simulink model "ssc_dcmtr_sl"  (R2022b)
settings: Solver=VariableStepAuto  StartTime=0.0  StopTime=10.0  RelTol=1e-3
model workspace (MAT data in the model file):
  J = 0.0946866703633
  K = 0.477771340295
  L = 0.000316454712175
  R = 4.99938152603
  Tbrk = 0.001
  Tcolumb = 0.001
  Ts = 0.01
  Tvis = 0.001
  b = 0.921434142151
libraries: fl_lib x6, nesl_utility x3, ee_lib x1
settings Model: Creator=smuckati  LastModifiedBy=smuckati
settings DebuggingCC: ParameterPrecisionLossMsg=none  UnconnectedInputMsg=warning  UnconnectedOutputMsg=warning  UnconnectedLineMsg=warning
settings ModelReferenceCC: EnableRefExpFcnMdlSchedulingChecks=on
settings RTWCC: DLArmComputeVersion=19.05

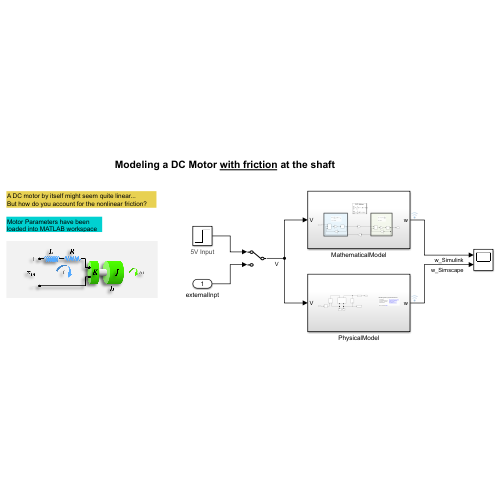
[thumbnail: Simulink's stored preview of the top-level diagram]
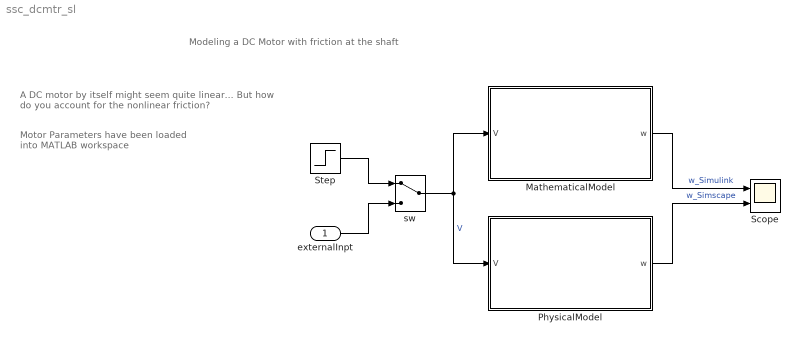
== system ssc_dcmtr_sl ==
  note: A DC motor by itself might seem quite linear...
      | But how do you account for the nonlinear friction?
  note: Modeling a DC Motor with friction at the shaft
  note: Motor Parameters have been loaded into MATLAB workspace
  externalInpt : Inport
  MathematicalModel : Subsystem
  PhysicalModel : Subsystem
  Scope : Scope  NumInputPorts=2
  Step : Step  Time=2  After=5  SampleTime=0
      settings: AttributesFormatString=5V Input
  sw : ManualSwitch
  wires:
  PhysicalModel/1(w) -> Scope/2  "w_Simscape"
  MathematicalModel/1(w) -> Scope/1  "w_Simulink"
  sw/1 -> PhysicalModel/1(V), MathematicalModel/1(V)  "V"
  externalInpt/1 -> sw/2
  Step/1 -> sw/1

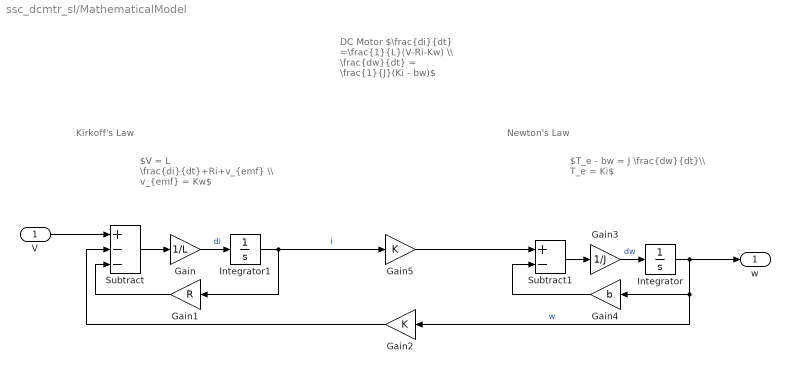
== system ssc_dcmtr_sl/MathematicalModel ==
  note: Newton's Law
  note: $T_e - bw = J \frac{dw}{dt}\\ T_e = Ki$
  note: Kirkoff's Law
  note: $V = L \frac{di}{dt}+Ri+v_{emf} \\ v_{emf} = Kw$
  note: DC Motor
      | $\frac{di}{dt} =\frac{1}{L}(V-Ri-Kw) \\ \frac{dw}{dt} = \frac{1}{J}(Ki - bw)$
  V : Inport
  Gain : Gain  Gain=1/L
  Gain1 : Gain  Gain=R
  Gain2 : Gain  Gain=K
  Gain3 : Gain  Gain=1/J
  Gain4 : Gain  Gain=b
  Gain5 : Gain  Gain=K
  Integrator : Integrator
  Integrator1 : Integrator
  Subtract : Sum  Inputs=+--
  Subtract1 : Sum  Inputs=+-
  w : Outport  VectorParamsAs1DForOutWhenUnconnected=off
  wires:
  Gain1/1 -> Subtract/3
  Integrator1/1 -> Gain5/1, Gain1/1  "i"
  Integrator/1 -> w/1, Gain2/1, Gain4/1  "w"
  Gain2/1 -> Subtract/2
  Subtract1/1 -> Gain3/1
  Gain3/1 -> Integrator/1  "dw"
  Gain4/1 -> Subtract1/2
  Gain5/1 -> Subtract1/1
  Subtract/1 -> Gain/1
  Gain/1 -> Integrator1/1  "di"
  V/1 -> Subtract/1

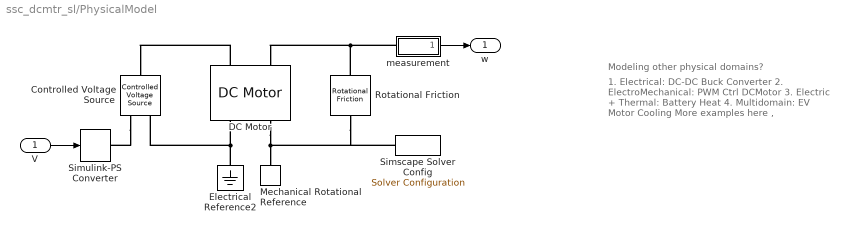
== system ssc_dcmtr_sl/PhysicalModel ==
  note: 1. Electrical: DC-DC Buck Converter
      | 2. ElectroMechanical: PWM Ctrl DCMotor
      | 3. Electric + Thermal: Battery Heat
      | 4. Multidomain: EV Motor Cooling
      |
      | More examples here ,
  note: Modeling other physical domains?
  V : Inport
  Controlled Voltage Source : fl_lib/Electrical/Electrical Sources/Controlled Voltage Source
  DC Motor : ee_lib/Electromechanical/Brushed Motors/DC Motor  field_option=ee.enum.field_option.pm  Rf=100 Ohm  Lf=1 H  Laf=0.15 H  If0=0 A  parameterization=ee.enum.dcparam_option.circuit_param  Ra=R Ohm  La=L H  emf_or_torque=ee.enum.emf_or_torque.ki  Kv=K V/(rad/s)  Ki=K N*m/A  T_stall=57/16 in*lbf  w_max=62.5 rpm  w_rated=1.5e+04 rpm  P_rated=0.08 W  V_rated=5 V  lam_param=ee.enum.lam_param.damping  i_noload=0 A  V_i_noload=1.5 V  J=J kg*m^2  lam=b N*m/(rad/s)  speed0=0 rpm  enable_fault_armature=simscape.enum.onoff.off  rev_faulted=1 / 3  G_faulted_armature=1e-5 S  fault_trigger_armature=ee.enum.faults.faultTrigger.temporal  t_fault_armature=1 s  max_permissible_current_armature=inf A  t_fail_on_current_armature=1 s  enable_fault_field=simscape.enum.onoff.off  G_faulted_field=1e-5 S  fault_trigger_field=ee.enum.faults.faultTrigger.temporal  t_fault_field=1 s  max_permissible_current_field=inf A  t_fail_on_current_field=1 s  fault_action=simscape.enum.assert.action.none  alpha=3.93e-3 1/K  Tmeas=25 degC  thermal_mass=100 J/K  initial_temperature=25 degC
  Electrical Reference2 : fl_lib/Electrical/Electrical Elements/Electrical Reference
  Mechanical Rotational Reference : fl_lib/Mechanical/Rotational Elements/Mechanical Rotational Reference
  Rotational Friction : fl_lib/Mechanical/Rotational Elements/Rotational Friction  brkwy_trq=Tbrk N*m  brkwy_vel=0.001 rad/s  Col_trq=Tcolumb N*m  visc_coef=Tvis N*m/(rad/s)  w_specify=off  w_priority=None  w=0 rad/s  w_nominal_specify=off  w_nominal_unit=rad/s  w_nominal_value=1  t_specify=off  t_priority=None  t=0 N*m  t_nominal_specify=off  t_nominal_unit=N*m  t_nominal_value=1
  Simscape Solver Config : nesl_utility/Solver Configuration  PhysicalDomain=network_engine_domain  SubClassName=solver  LeftPortType=input  RightPortType=generic  Tones=[]  Harmonics=[]  SimulateNoise=off  Profile=off  UseLocalSampling=off  EnableSwitchedLinearOptims=on  FrequencyDomain=off  UseCCode=off  RelTol=0.001  AbsTol=1e-06  MinStep=1e-09  ToWorkspace=off  RevertToSquareIcSolve=off  NumHomotopyIterations=100  PhasorMode=off  PhasorModeNumHarmonics=1  ConsistencySolver=NEWTON_XTOL_AFTER_FTOL  IndexReductionMethod=DerivativeReplacement  DoDC=off  ResidualTolerance=1e-9  ConsistencyTolSource=GLOBAL  ConsistencyAbsTol=0.001  ConsistencyRelTol=0.001  ConsistencyTolFactor=0.001  UseLocalSolver=off  LocalSolverChoice=NE_BACKWARD_EULER_ADVANCER  ResolveIndetEquations=on  FunctionEvalNumThread=1  LocalSolverSampleTime=0.00125  DoFixedCost=off  MaxNonlinIter=3  MaxModeIter=2  ComputeImpulses=off  ImpulseIterations=2  LinearAlgebra=Sparse  LinearAlgebraNumThread=0  EquationFormulation=NE_TIME_EF  DelaysMemoryBudget=1024  AutomaticFiltering=on  FilteringTimeConstant=0.001  PartitionStorageMethod=AS_NEEDED  PartitionMemoryBudget=1024  PartitionMethod=FAST
  Simulink-PS Converter : nesl_utility/Simulink-PS Converter  PhysicalDomain=network_engine_domain  SubClassName=ps_input  LeftPortType=input  RightPortType=output  PseudoPeriodic=off  Frequencies=[]  NoiseDistribution=none  NoiseParameters=[]  Unit=1  AffineConversion=off  FilteringAndDerivatives=zero  SimscapeFilterOrder=1  InputFilterTimeConstant=.001  UdotUserProvided=0
  measurement : Subsystem
      settings: PortSchema="{\"entries\":[{\"content\":{\"sides\":[{\"content\":{\"connectorIds\":[]},\"type\":\"ConnectorPlacement.EquallySpacedRectSide\",\"uuid\":\"abba8c98-b5a4-4c4c-8426-d04bb5bd8376\"},{\"content\":{\"connectorIds\":[],\"side\":\"RIGHT\"},\"type\":\"ConnectorPlacement.EquallySpacedRectSide\",\"uuid\":\"4c88a845-695e-489f-8958-399be31258ba\"},{\"content\":{\"connectorIds\":[\"LConn1\"],\"side\":\"TOP\"},\"type\":\"ConnectorPlacement.EquallySpacedRectSide\",\"uuid\":\"679bc764-0dc4-40d2-b029-a4ea74e3efc8\"},{\"content\":{\"connectorIds\":[\"Out1\"],\"side\":\"BOTTOM\"},\"type\":\"ConnectorPlacement.EquallySpacedRectSide\",\"uuid\":\"9fb1c662-f4af-4578-8c70-f395a6f7f535\"}]},\"type\":\"ConnectorPlacement.EquallySpacedConnector\",\"uuid\":\"424eb965-f1ce-46f3-b179-04fc10bc201b\"}],\"packageUris\":[\"http://schema.mathworks.com/mf0/Connector/R2020b\"],\"version\":\"1.0\"}"
      mask Display: disp('Sensor')
  w : Outport  VectorParamsAs1DForOutWhenUnconnected=off
  wires:
  V/1 -> Simulink-PS Converter/1
  measurement/1(ang_vel) -> w/1
  connections:
  Electrical Reference2/LConn1 -- Controlled Voltage Source/RConn2 -- DC Motor/RConn1
  Controlled Voltage Source/RConn1 -- Simulink-PS Converter/RConn1
  DC Motor/RConn2 -- Rotational Friction/RConn1 -- Simscape Solver Config/RConn1 -- Mechanical Rotational Reference/LConn1
  measurement/LConn1 -- Rotational Friction/LConn1 -- DC Motor/LConn2
  DC Motor/LConn1 -- Controlled Voltage Source/LConn1

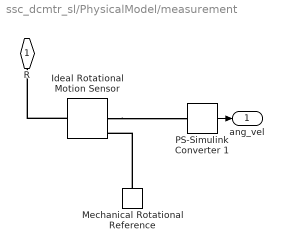
== system ssc_dcmtr_sl/PhysicalModel/measurement ==
  Ideal Rotational Motion Sensor : fl_lib/Mechanical/Mechanical Sensors/Ideal Rotational Motion Sensor  reference=foundation.enum.MeasurementReference.difference  acceleration_port=false  velocity_port=true  position_port=true  wrap_angle=simscape.enum.onoff.off  offset=0 rad
  Mechanical Rotational Reference : fl_lib/Mechanical/Rotational Elements/Mechanical Rotational Reference
  PS-Simulink Converter 1 : nesl_utility/PS-Simulink Converter  PhysicalDomain=network_engine_domain  SubClassName=ps_output  LeftPortType=input  RightPortType=output  PseudoPeriodic=off  Frequencies=[]  VectorFormat=1-D array  Unit=rad/s  AffineConversion=off
  R : PMIOPort  Side=Left
  ang_vel : Outport
  wires:
  PS-Simulink Converter 1/1 -> ang_vel/1
  connections:
  Ideal Rotational Motion Sensor/RConn2 -- PS-Simulink Converter 1/LConn1
  Mechanical Rotational Reference/LConn1 -- Ideal Rotational Motion Sensor/RConn1
  Ideal Rotational Motion Sensor/LConn1 -- R/RConn1
